simulink model "sm_stewart_platform"  (R2019b)
settings: Solver=ode45  StartTime=0.0  StopTime=450  MaxStep=0.2  RelTol=1e-3  EnableMultiTasking=on
model workspace (MAT data in the model file):
  g_density = 5
values from neighbouring files (symbols this model uses):
  B = base_points.Data(:,:,1)    [run_this_for_sim.m]
  base_radius = 0.75*100    (= 75)    [run_this_for_sim.m]
  desired_max_angle = 10    [run_this_for_sim.m]
  desired_max_x = 0.05    [run_this_for_sim.m]
  desired_max_y = desired_max_x    (= 0.05)    [run_this_for_sim.m]
  desired_max_z = 0.05    [run_this_for_sim.m]
  initial_integral_force = 200    [run_this_for_sim.m]
  leg_max = leg_min+0.3    (= 1.322)    [run_this_for_sim.m]
  leg_min = 1.022    [run_this_for_sim.m]
  leg_thickness = 75/1000    (= 0.075)    [run_this_for_sim.m]
  lower_leg_length = upper_leg_length    (= 0.511)    [run_this_for_sim.m]
  max_velocity = 0.15    [run_this_for_sim.m]
  P = platform_points.Data(:,:,1)    [run_this_for_sim.m]
  platform_radius = 0.75*base_radius    (= 56.25)    [run_this_for_sim.m]
  platform_thickness = 0.1/8    (= 0.0125)    [run_this_for_sim.m]
  trajectory_smoothing = 1/1.5    (= 0.666666666667)    [run_this_for_sim.m]
  upper_leg_length = dead_length/2    (= 0.511)    [run_this_for_sim.m]
  work_height = 1.2*100    (= 120)    [run_this_for_sim.m]
undefined symbols (not defined in the file or in its folder): nom_length, X, Z
libraries: sp_lib x18, nesl_utility x11, sm_lib x9, simulink x2
(part 4 of 10)

== system sm_stewart_platform/Reference Trajectory Generator6/Euler XYZ ==
  angles : Inport
  11 : Fcn  Expr=cos(u[2])*cos(u[3])
  12 : Fcn  Expr=-cos(u[2])*sin(u[3])
  13 : Fcn  Expr=sin(u[2])
  21 : Fcn  Expr=cos(u[3])*sin(u[2])*sin(u[1])+cos(u[1])*sin(u[3])
  22 : Fcn  Expr=cos(u[1])*cos(u[3]) - sin(u[1])*sin(u[2])*sin(u[3])
  23 : Fcn  Expr=-sin(u[1])*cos(u[2])
  31 : Fcn  Expr=sin(u[1])*sin(u[3]) - cos(u[1])*cos(u[3])*sin(u[2])
  32 : Fcn  Expr=cos(u[3])*sin(u[1])+cos(u[1])*sin(u[2])*sin(u[3])
  33 : Fcn  Expr=cos(u[1])*cos(u[2])
  Mux2 : Mux  Inputs=9
  Reshape 9x1->3x3 : Reshape  OutputDimensionality=Customize  OutputDimensions=[3,3]
  R : Outport  VectorParamsAs1DForOutWhenUnconnected=off
  wires:
  angles/1 -> 23/1, 33/1, 13/1, 32/1, 22/1, 12/1, 31/1, 21/1, 11/1
  33/1 -> Mux2/9
  23/1 -> Mux2/8
  13/1 -> Mux2/7
  32/1 -> Mux2/6
  22/1 -> Mux2/5
  12/1 -> Mux2/4
  31/1 -> Mux2/3
  21/1 -> Mux2/2
  11/1 -> Mux2/1
  Mux2/1 -> Reshape 9x1->3x3/1
  Reshape 9x1->3x3/1 -> R/1

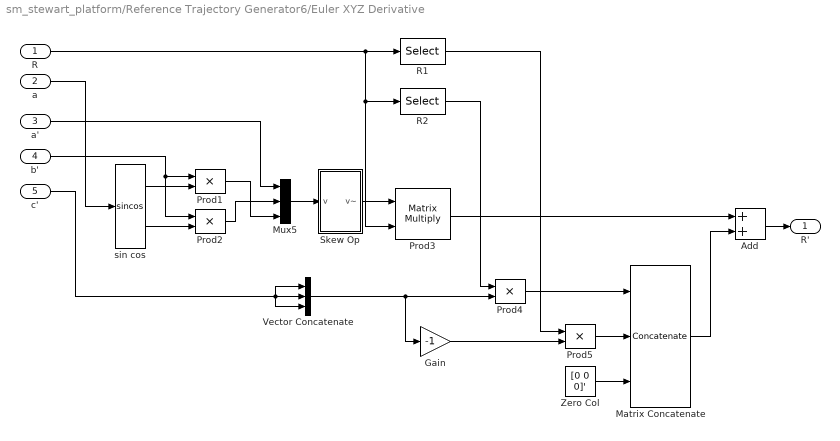
== system sm_stewart_platform/Reference Trajectory Generator6/Euler XYZ Derivative ==
  R : Inport
  a : Inport  Port=2
  a' : Inport  Port=3
  b' : Inport  Port=4
  c' : Inport  Port=5
  Add : Sum
  Gain : Gain  Gain=-1
  Matrix Concatenate : Concatenate  NumInputs=3  Mode=Multidimensional array  ConcatenateDimension=2
  Mux5 : Mux  Inputs=3
  Prod{1..2,4..5} (4 alike) : Product  RndMeth=Zero
  Prod3 : Product  Multiplication=Matrix(*)  RndMeth=Zero
  R1 : Selector  NumberOfDimensions=2  InputPortWidth=3  IndexOptions=Select all,Index vector (dialog)  Indices=[1 3],1  OutputSizes=1,1
  R2 : Selector  NumberOfDimensions=2  InputPortWidth=3  IndexOptions=Select all,Index vector (dialog)  Indices=[1 3],2  OutputSizes=1,1
  Skew Op : Subsystem
  Vector Concatenate : Concatenate  NumInputs=3  Mode=Multidimensional array
  Zero Col : Constant  Value=[0 0 0]'
  sin cos : Trigonometry  Operator=sincos
  R' : Outport  VectorParamsAs1DForOutWhenUnconnected=off
  wires:
  a/1 -> sin cos/1
  sin cos/1 -> Prod1/2
  sin cos/2 -> Prod2/2
  b'/1 -> Prod2/1, Prod1/1
  a'/1 -> Mux5/1
  Prod2/1 -> Mux5/2
  Prod1/1 -> Mux5/3
  Mux5/1 -> Skew Op/1(v)
  Vector Concatenate/1 -> Prod4/2, Gain/1
  R2/1 -> Prod4/1
  Gain/1 -> Prod5/2
  Zero Col/1 -> Matrix Concatenate/3
  Prod5/1 -> Matrix Concatenate/2
  Prod4/1 -> Matrix Concatenate/1
  R1/1 -> Prod5/1
  Prod3/1 -> Add/1
  Matrix Concatenate/1 -> Add/2
  Add/1 -> R'/1
  R/1 -> R1/1, Prod3/2, R2/1
  Skew Op/1(v~) -> Prod3/1
  c'/1 -> Vector Concatenate/2, Vector Concatenate/1, Vector Concatenate/3

== system sm_stewart_platform/Reference Trajectory Generator6/Rx sinusoid ==
  t : Inport
  Add : Sum  Inputs=|++
  Add2 : Sum  Inputs=++|
  amp1 : Gain  Gain=A
  amp2 : Gain  Gain=w*A*pi/180
  deg2rad : Gain  Gain=pi/180
  freq : Gain  Gain=w
  offset : Constant  Value=k  VectorParams1D=off
  phase : Constant  Value=p  VectorParams1D=off
  sin cos : Trigonometry  Operator=sincos
  f : Outport  VectorParamsAs1DForOutWhenUnconnected=off
  f' : Outport  Port=2  VectorParamsAs1DForOutWhenUnconnected=off
  wires:
  t/1 -> freq/1
  Add/1 -> deg2rad/1
  phase/1 -> Add/2
  amp2/1 -> f'/1
  Add2/1 -> f/1
  offset/1 -> Add2/1
  sin cos/1 -> amp1/1
  sin cos/2 -> amp2/1
  amp1/1 -> Add2/2
  freq/1 -> Add/1
  deg2rad/1 -> sin cos/1

== system sm_stewart_platform/Reference Trajectory Generator6/Ry sinusoid ==
  t : Inport
  Add : Sum  Inputs=|++
  Add2 : Sum  Inputs=++|
  amp1 : Gain  Gain=A
  amp2 : Gain  Gain=w*A*pi/180
  deg2rad : Gain  Gain=pi/180
  freq : Gain  Gain=w
  offset : Constant  Value=k  VectorParams1D=off
  phase : Constant  Value=p  VectorParams1D=off
  sin cos : Trigonometry  Operator=sincos
  f : Outport  VectorParamsAs1DForOutWhenUnconnected=off
  f' : Outport  Port=2  VectorParamsAs1DForOutWhenUnconnected=off
  wires:
  t/1 -> freq/1
  Add/1 -> deg2rad/1
  phase/1 -> Add/2
  amp2/1 -> f'/1
  Add2/1 -> f/1
  offset/1 -> Add2/1
  sin cos/1 -> amp1/1
  sin cos/2 -> amp2/1
  amp1/1 -> Add2/2
  freq/1 -> Add/1
  deg2rad/1 -> sin cos/1

== system sm_stewart_platform/Reference Trajectory Generator6/Rz sinusoid ==
  t : Inport
  Add : Sum  Inputs=|++
  Add2 : Sum  Inputs=++|
  amp1 : Gain  Gain=A
  amp2 : Gain  Gain=w*A*pi/180
  deg2rad : Gain  Gain=pi/180
  freq : Gain  Gain=w
  offset : Constant  Value=k  VectorParams1D=off
  phase : Constant  Value=p  VectorParams1D=off
  sin cos : Trigonometry  Operator=sincos
  f : Outport  VectorParamsAs1DForOutWhenUnconnected=off
  f' : Outport  Port=2  VectorParamsAs1DForOutWhenUnconnected=off
  wires:
  t/1 -> freq/1
  Add/1 -> deg2rad/1
  phase/1 -> Add/2
  amp2/1 -> f'/1
  Add2/1 -> f/1
  offset/1 -> Add2/1
  sin cos/1 -> amp1/1
  sin cos/2 -> amp2/1
  amp1/1 -> Add2/2
  freq/1 -> Add/1
  deg2rad/1 -> sin cos/1

== system sm_stewart_platform/Reference Trajectory Generator6/dx sinusoid ==
  t : Inport
  Add : Sum  Inputs=|++
  Add2 : Sum  Inputs=++|
  amp1 : Gain  Gain=A
  amp2 : Gain  Gain=w*A*pi/180
  deg2rad : Gain  Gain=pi/180
  freq : Gain  Gain=w
  offset : Constant  Value=k  VectorParams1D=off
  phase : Constant  Value=p  VectorParams1D=off
  sin cos : Trigonometry  Operator=sincos
  f : Outport  VectorParamsAs1DForOutWhenUnconnected=off
  f' : Outport  Port=2  VectorParamsAs1DForOutWhenUnconnected=off
  wires:
  t/1 -> freq/1
  Add/1 -> deg2rad/1
  phase/1 -> Add/2
  amp2/1 -> f'/1
  Add2/1 -> f/1
  offset/1 -> Add2/1
  sin cos/1 -> amp1/1
  sin cos/2 -> amp2/1
  amp1/1 -> Add2/2
  freq/1 -> Add/1
  deg2rad/1 -> sin cos/1

== system sm_stewart_platform/Reference Trajectory Generator6/dy sinusoid ==
  t : Inport
  Add : Sum  Inputs=|++
  Add2 : Sum  Inputs=++|
  amp1 : Gain  Gain=A
  amp2 : Gain  Gain=w*A*pi/180
  deg2rad : Gain  Gain=pi/180
  freq : Gain  Gain=w
  offset : Constant  Value=k  VectorParams1D=off
  phase : Constant  Value=p  VectorParams1D=off
  sin cos : Trigonometry  Operator=sincos
  f : Outport  VectorParamsAs1DForOutWhenUnconnected=off
  f' : Outport  Port=2  VectorParamsAs1DForOutWhenUnconnected=off
  wires:
  t/1 -> freq/1
  Add/1 -> deg2rad/1
  phase/1 -> Add/2
  amp2/1 -> f'/1
  Add2/1 -> f/1
  offset/1 -> Add2/1
  sin cos/1 -> amp1/1
  sin cos/2 -> amp2/1
  amp1/1 -> Add2/2
  freq/1 -> Add/1
  deg2rad/1 -> sin cos/1

== system sm_stewart_platform/Reference Trajectory Generator6/dz sinusoid ==
  t : Inport
  Add : Sum  Inputs=|++
  Add2 : Sum  Inputs=++|
  amp1 : Gain  Gain=A
  amp2 : Gain  Gain=w*A*pi/180
  deg2rad : Gain  Gain=pi/180
  freq : Gain  Gain=w
  offset : Constant  Value=k  VectorParams1D=off
  phase : Constant  Value=p  VectorParams1D=off
  sin cos : Trigonometry  Operator=sincos
  f : Outport  VectorParamsAs1DForOutWhenUnconnected=off
  f' : Outport  Port=2  VectorParamsAs1DForOutWhenUnconnected=off
  wires:
  t/1 -> freq/1
  Add/1 -> deg2rad/1
  phase/1 -> Add/2
  amp2/1 -> f'/1
  Add2/1 -> f/1
  offset/1 -> Add2/1
  sin cos/1 -> amp1/1
  sin cos/2 -> amp2/1
  amp1/1 -> Add2/2
  freq/1 -> Add/1
  deg2rad/1 -> sin cos/1

== system sm_stewart_platform/Reference Trajectory Generator6/manual ==
  Constant : Constant
  Constant1 : Constant  Value=work_height
  Derivative : Derivative
  Slider Gain : simulink/Math Operations/Slider Gain  gain=-45.0  low=-250  high=250
  Sum : Sum  Inputs=|++
  x : Outport  VectorParamsAs1DForOutWhenUnconnected=off
  x' : Outport  Port=2  VectorParamsAs1DForOutWhenUnconnected=off
  wires:
  Sum/1 -> Derivative/1, x/1
  Constant/1 -> Slider Gain/1
  Derivative/1 -> x'/1
  Slider Gain/1 -> Sum/1
  Constant1/1 -> Sum/2

== system sm_stewart_platform/Stewart Platform System/Controller ==
  act_pos : Inport
  act_vel : Inport  Port=2
  des_pos : Inport  Port=3
  des_vel : Inport  Port=4
  D : Gain  Gain=Kd  SaturateOnIntegerOverflow=on  OutDataTypeStr=Inherit: Same as input  ParamDataTypeStr=Inherit: Same as input
  Gain : Gain
  I : Gain  Gain=Ki  SaturateOnIntegerOverflow=on  OutDataTypeStr=Inherit: Same as input  ParamDataTypeStr=Inherit: Same as input
  Integrator : Integrator  InitialCondition=initial_integral_force/Ki(1)
  P : Gain  Gain=Kp  SaturateOnIntegerOverflow=on  OutDataTypeStr=Inherit: Same as input  ParamDataTypeStr=Inherit: Same as input
  PID : Scope  NumInputPorts=3
  Sum : Sum  Inputs=-+|  SaturateOnIntegerOverflow=on  InputSameDT=on  OutDataTypeStr=Inherit: Same as first input
  Sum1 : Sum  Inputs=+++  SaturateOnIntegerOverflow=on  InputSameDT=on  OutDataTypeStr=Inherit: Same as first input
  Sum2 : Sum  Inputs=-+|  SaturateOnIntegerOverflow=on  InputSameDT=on  OutDataTypeStr=Inherit: Same as first input
  force : Outport  VectorParamsAs1DForOutWhenUnconnected=off
  wires:
  Sum/1 -> Integrator/1, P/1
  P/1 -> PID/1, Sum1/1
  act_pos/1 -> Sum/1
  des_pos/1 -> Sum/2
  act_vel/1 -> Sum2/1
  des_vel/1 -> Gain/1
  D/1 -> PID/3, Sum1/3
  I/1 -> PID/2, Sum1/2
  Sum1/1 -> force/1
  Integrator/1 -> I/1
  Gain/1 -> Sum2/2
  Sum2/1 -> D/1

== system sm_stewart_platform/Stewart Platform System/Ideal PID ==
  act_pos : Inport
  act_vel : Inport  Port=2
  des_pos : Inport  Port=3
  des_vel : Inport  Port=4
  D : Gain  Gain=Kd  SaturateOnIntegerOverflow=on  OutDataTypeStr=Inherit: Same as input  ParamDataTypeStr=Inherit: Same as input
  Gain : Gain
  I : Gain  Gain=1/Ki  SaturateOnIntegerOverflow=on  OutDataTypeStr=Inherit: Same as input  ParamDataTypeStr=Inherit: Same as input
  Ideal PID : Scope  NumInputPorts=3
  Integrator : Integrator  InitialCondition=initial_integral_force*Ki(1)/Kp(1)
  P{,1..3} (4 alike) : Gain  Gain=Kp  SaturateOnIntegerOverflow=on  OutDataTypeStr=Inherit: Same as input  ParamDataTypeStr=Inherit: Same as input
  Sum : Sum  Inputs=-+|  SaturateOnIntegerOverflow=on  InputSameDT=on  OutDataTypeStr=Inherit: Same as first input
  Sum1 : Sum  Inputs=+++  SaturateOnIntegerOverflow=on  InputSameDT=on  OutDataTypeStr=Inherit: Same as first input
  Sum2 : Sum  Inputs=-+|  SaturateOnIntegerOverflow=on  InputSameDT=on  OutDataTypeStr=Inherit: Same as first input
  force : Outport  VectorParamsAs1DForOutWhenUnconnected=off
  wires:
  Sum/1 -> P1/1, Sum1/1, Integrator/1
  act_pos/1 -> Sum/1
  des_pos/1 -> Sum/2
  act_vel/1 -> Sum2/1
  des_vel/1 -> Gain/1
  Integrator/1 -> I/1
  Gain/1 -> Sum2/2
  P/1 -> force/1
  I/1 -> P2/1, Sum1/2
  D/1 -> P3/1, Sum1/3
  Sum1/1 -> P/1
  P1/1 -> Ideal PID/1
  P2/1 -> Ideal PID/2
  P3/1 -> Ideal PID/3
  Sum2/1 -> D/1

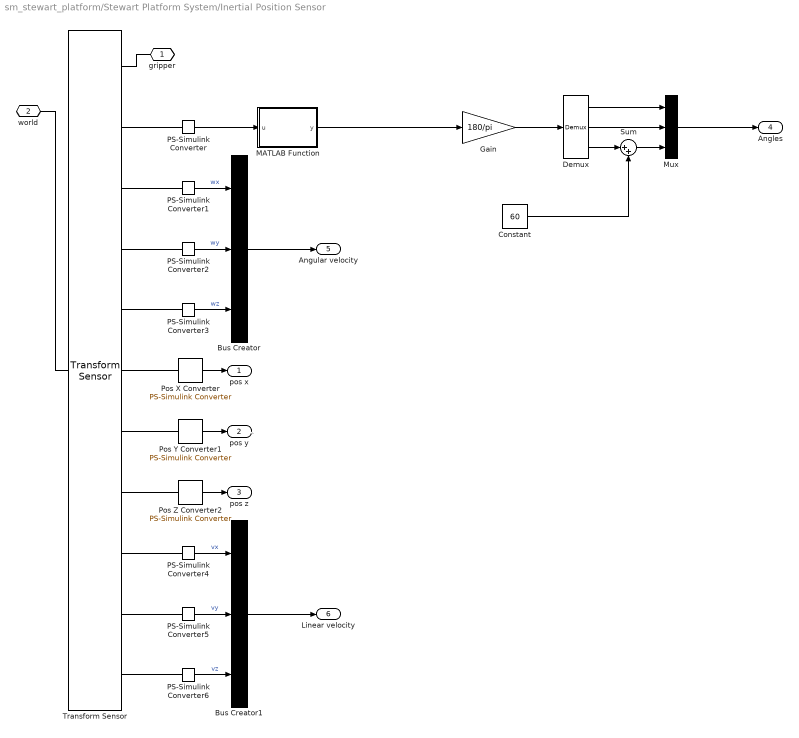
== system sm_stewart_platform/Stewart Platform System/Inertial Position Sensor ==
  note: `
  Bus Creator : BusCreator  Inputs=3
  Bus Creator1 : BusCreator  Inputs=3
  Constant : Constant  Value=60
  Demux : Demux  Outputs=3
  Gain : Gain  Gain=180/pi
  MATLAB Function : MATLAB Function  TreatAsAtomicUnit=on
  Mux : Mux  Inputs=3
  PS-Simulink Converter : nesl_utility/PS-Simulink Converter  PhysicalDomain=network_engine_domain  SubClassName=ps_output  LeftPortType=input  RightPortType=output  PseudoPeriodic=off  Frequencies=[]  Unit=1  AffineConversion=off
  PS-Simulink Converter1 : nesl_utility/PS-Simulink Converter  PhysicalDomain=network_engine_domain  SubClassName=ps_output  LeftPortType=input  RightPortType=output  PseudoPeriodic=off  Frequencies=[]  Unit=deg/s  AffineConversion=off
  PS-Simulink Converter2 : nesl_utility/PS-Simulink Converter  PhysicalDomain=network_engine_domain  SubClassName=ps_output  LeftPortType=input  RightPortType=output  PseudoPeriodic=off  Frequencies=[]  Unit=deg/s  AffineConversion=off
  PS-Simulink Converter3 : nesl_utility/PS-Simulink Converter  PhysicalDomain=network_engine_domain  SubClassName=ps_output  LeftPortType=input  RightPortType=output  PseudoPeriodic=off  Frequencies=[]  Unit=deg/s  AffineConversion=off
  PS-Simulink Converter4 : nesl_utility/PS-Simulink Converter  PhysicalDomain=network_engine_domain  SubClassName=ps_output  LeftPortType=input  RightPortType=output  PseudoPeriodic=off  Frequencies=[]  Unit=m/s  AffineConversion=off
  PS-Simulink Converter5 : nesl_utility/PS-Simulink Converter  PhysicalDomain=network_engine_domain  SubClassName=ps_output  LeftPortType=input  RightPortType=output  PseudoPeriodic=off  Frequencies=[]  Unit=m/s  AffineConversion=off
  PS-Simulink Converter6 : nesl_utility/PS-Simulink Converter  PhysicalDomain=network_engine_domain  SubClassName=ps_output  LeftPortType=input  RightPortType=output  PseudoPeriodic=off  Frequencies=[]  Unit=m/s  AffineConversion=off
  Pos X Converter : nesl_utility/PS-Simulink Converter  PhysicalDomain=network_engine_domain  SubClassName=ps_output  LeftPortType=input  RightPortType=output  PseudoPeriodic=off  Frequencies=[]  Unit=cm  AffineConversion=off
  Pos Y Converter1 : nesl_utility/PS-Simulink Converter  PhysicalDomain=network_engine_domain  SubClassName=ps_output  LeftPortType=input  RightPortType=output  PseudoPeriodic=off  Frequencies=[]  Unit=cm  AffineConversion=off
  Pos Z Converter2 : nesl_utility/PS-Simulink Converter  PhysicalDomain=network_engine_domain  SubClassName=ps_output  LeftPortType=input  RightPortType=output  PseudoPeriodic=off  Frequencies=[]  Unit=cm  AffineConversion=off
  Sum : Sum  Inputs=|++
  Transform Sensor : sm_lib/Frames and Transforms/Transform Sensor  MeasurementFrame=World  SenseAngle=off  SenseAxis=off  SenseAngle1=off  SenseAngle2=off  SenseAngle3=off  SenseQ=on  SenseR=off  SenseOmegaX=on  SenseOmegaY=on  SenseOmegaZ=on  SenseOmega1=off  SenseOmega2=off  SenseOmega3=off  SenseQDot=off  SenseRDot=off  SenseAlphaX=off  SenseAlphaY=off  SenseAlphaZ=off  SenseAlpha1=off  SenseAlpha2=off  SenseAlpha3=off  SenseQDDot=off  SenseRDDot=off  SenseX=on  SenseY=on  SenseZ=on  SenseRad=off  SenseAzim=off  SenseDist=off  SenseInc=off  SenseXDot=on  SenseYDot=on  SenseZDot=on  SenseRadDot=off  SenseAzimDot=off  SenseDistDot=off  SenseIncDot=off  SenseXDDot=off  SenseYDDot=off  SenseZDDot=off  SenseRadDDot=off  SenseAzimDDot=off  SenseDistDDot=off  SenseIncDDot=off
  gripper : PMIOPort  Side=Left
  world : PMIOPort  Port=2  Side=Left
  pos x : Outport  VectorParamsAs1DForOutWhenUnconnected=off
  pos y : Outport  Port=2  VectorParamsAs1DForOutWhenUnconnected=off
  pos z : Outport  Port=3  VectorParamsAs1DForOutWhenUnconnected=off
  Angles : Outport  Port=4  VectorParamsAs1DForOutWhenUnconnected=off
  Angular velocity : Outport  Port=5  VectorParamsAs1DForOutWhenUnconnected=off
  Linear velocity : Outport  Port=6  VectorParamsAs1DForOutWhenUnconnected=off
  wires:
  Pos Z Converter2/1 -> pos z/1
  Pos Y Converter1/1 -> pos y/1
  Pos X Converter/1 -> pos x/1
  PS-Simulink Converter/1 -> MATLAB Function/1(u)
  MATLAB Function/1(y) -> Gain/1
  Gain/1 -> Demux/1
  Demux/1 -> Mux/1
  Demux/2 -> Mux/2
  Mux/1 -> Angles/1
  Demux/3 -> Sum/1
  Sum/1 -> Mux/3
  Constant/1 -> Sum/2
  PS-Simulink Converter1/1 -> Bus Creator/1  "wx"
  PS-Simulink Converter2/1 -> Bus Creator/2  "wy"
  PS-Simulink Converter3/1 -> Bus Creator/3  "wz"
  PS-Simulink Converter4/1 -> Bus Creator1/1  "vx"
  PS-Simulink Converter6/1 -> Bus Creator1/3  "vz"
  PS-Simulink Converter5/1 -> Bus Creator1/2  "vy"
  Bus Creator/1 -> Angular velocity/1
  Bus Creator1/1 -> Linear velocity/1
  connections:
  world/RConn1 -- Transform Sensor/LConn1
  gripper/RConn1 -- Transform Sensor/RConn1
  PS-Simulink Converter/LConn1 -- Transform Sensor/RConn2
  Pos X Converter/LConn1 -- Transform Sensor/RConn6
  Transform Sensor/RConn7 -- Pos Y Converter1/LConn1
  Transform Sensor/RConn8 -- Pos Z Converter2/LConn1
  PS-Simulink Converter1/LConn1 -- Transform Sensor/RConn3
  Transform Sensor/RConn4 -- PS-Simulink Converter2/LConn1
  PS-Simulink Converter3/LConn1 -- Transform Sensor/RConn5
  Transform Sensor/RConn9 -- PS-Simulink Converter4/LConn1
  Transform Sensor/RConn10 -- PS-Simulink Converter5/LConn1
  Transform Sensor/RConn11 -- PS-Simulink Converter6/LConn1

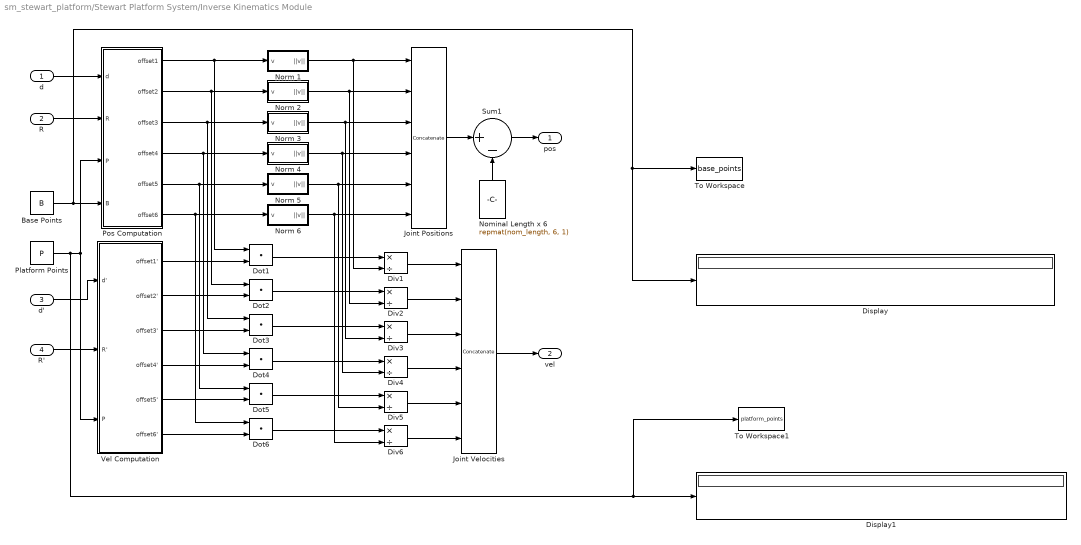
== system sm_stewart_platform/Stewart Platform System/Inverse Kinematics Module ==
  d : Inport
  R : Inport  Port=2
  d' : Inport  Port=3
  R' : Inport  Port=4
  Base Points : Constant  Value=B
  Display : Display
  Display1 : Display
  Div{1..6} (6 alike) : Product  Inputs=*/
  Dot{1..6} (6 alike) : DotProduct  OutDataTypeStr=Inherit: Inherit via internal rule
  Joint Positions : Concatenate  NumInputs=6  Mode=Multidimensional array
  Joint Velocities : Concatenate  NumInputs=6  Mode=Multidimensional array
  Nominal Length x 6 : Constant  Value=repmat(nom_length, 6, 1)
  Norm 1 : Subsystem
  Norm 2 : Subsystem
  Norm 3 : Subsystem
  Norm 4 : Subsystem
  Norm 5 : Subsystem
  Norm 6 : Subsystem
  Platform Points : Constant  Value=P
  Pos Computation : Subsystem
  Sum1 : Sum  Inputs=|+-
  To Workspace : ToWorkspace  VariableName=base_points  SaveFormat=Timeseries  SampleTime=-1
  To Workspace1 : ToWorkspace  VariableName=platform_points  SaveFormat=Timeseries  SampleTime=-1
  Vel Computation : Subsystem
  pos : Outport  VectorParamsAs1DForOutWhenUnconnected=off
  vel : Outport  Port=2  VectorParamsAs1DForOutWhenUnconnected=off
  wires:
  Joint Positions/1 -> Sum1/1
  Nominal Length x 6/1 -> Sum1/2
  Sum1/1 -> pos/1
  d/1 -> Pos Computation/1(d)
  R/1 -> Pos Computation/2(R)
  Base Points/1 -> To Workspace/1, Display/1, Pos Computation/4(B)
  Platform Points/1 -> To Workspace1/1, Display1/1, Vel Computation/3(P), Pos Computation/3(P)
  Pos Computation/4(offset4) -> Norm 4/1(v), Dot4/1
  Pos Computation/3(offset3) -> Norm 3/1(v), Dot3/1
  Pos Computation/2(offset2) -> Norm 2/1(v), Dot2/1
  Pos Computation/1(offset1) -> Norm 1/1(v), Dot1/1
  Pos Computation/5(offset5) -> Norm 5/1(v), Dot5/1
  Pos Computation/6(offset6) -> Norm 6/1(v), Dot6/1
  Norm 1/1(||v||) -> Joint Positions/1, Div1/2
  Norm 6/1(||v||) -> Joint Positions/6, Div6/2
  Norm 2/1(||v||) -> Joint Positions/2, Div2/2
  Norm 3/1(||v||) -> Joint Positions/3, Div3/2
  Norm 4/1(||v||) -> Joint Positions/4, Div4/2
  Norm 5/1(||v||) -> Joint Positions/5, Div5/2
  Vel Computation/3(offset3') -> Dot3/2
  Vel Computation/4(offset4') -> Dot4/2
  Vel Computation/2(offset2') -> Dot2/2
  Vel Computation/5(offset5') -> Dot5/2
  Vel Computation/6(offset6') -> Dot6/2
  d'/1 -> Vel Computation/1(d')
  Dot2/1 -> Div2/1
  Dot6/1 -> Div6/1
  Dot5/1 -> Div5/1
  Dot4/1 -> Div4/1
  Dot3/1 -> Div3/1
  Div1/1 -> Joint Velocities/1
  Div2/1 -> Joint Velocities/2
  Div6/1 -> Joint Velocities/6
  Div3/1 -> Joint Velocities/3
  Div4/1 -> Joint Velocities/4
  Div5/1 -> Joint Velocities/5
  Joint Velocities/1 -> vel/1
  R'/1 -> Vel Computation/2(R')
  Vel Computation/1(offset1') -> Dot1/2
  Dot1/1 -> Div1/1

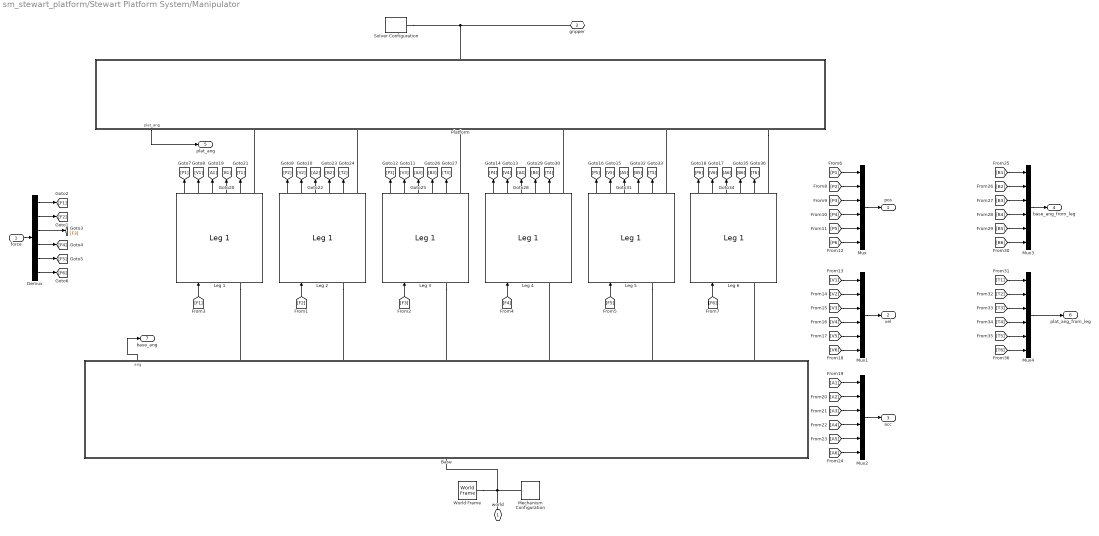
== system sm_stewart_platform/Stewart Platform System/Manipulator ==
  force : Inport
  Base : Subsystem  AncestorBlock=sm_stewart_platform_lib/Hexagon Plate  mask(Hexagon Plate){kind=base, hex_rad=base_rad, hex_thick=base_thick, hex_skew=hex_skew, flange_sep=2 * leg_rad * cos(pi/6) - flange_thick, flange_len=flange_len, flange_width=flange_width, flange_thick=flange_thick, diffuse=[0.4 0.3 0.2 0.5], specular=[0 0 0], shininess=10}
      mask prompts: hex_rad "Hexagon Radius (cm)"; hex_thick "Hexagon Thickness (cm)"; hex_skew "Hexagon Skew"; flange_sep "Flange Separation (cm)"; flange_len "Flange Length (cm)"; flange_width "Flange Width (cm)"; flange_thick "Flange Thickness (cm)"; diffuse "Diffuse (rgba)"; specular "Specular (rgba)"
      mask help:
      | Models a rigid body formed by attaching six couplings to the corners of a skewed hexagon.
      |
      | There are two hexagon plates in a Stewart platform manipulator: one forming the grounded base, and the other forming the moveable platform.  Six legs connect the corresponding couplings of these two plates.  Both plates are modeled with this block.
      mask init:
      | % Set up a value equal to 0 or 1 based on whether
      | % this is the base or platform, respectively.  This value
      | % is used in the computations of certain variables and
      | % transforms that differ for the two types of hexagon plates.
      | if (kind == 1)
      |     kind_val = 0;  % Value for base
      | else
      |     kind_val = 1;  % Value for platform
      | end
      mask Help:
      | A <em>Hexagon Plate</em> models a rigid body formed by attaching six couplings to the corners of a skewed hexagon.
      | 
      | There are two hexagon plates in a Stewart platform manipulator: one forming the grounded base, and the other forming the moveable platform.  Six legs connect the corresponding couplings of these two plates.  Both plates are modeled with this block.
      | 
      | <h3>Skewed Hexagons</h3>
      | 
      | The main part of a hexagon plate is a </em>skewed hexagon</em>.  This is short hexagonal prism.  The cross section is based on a regular hexagon, but with the vertices perturbed according to the skew factor, a real value in the range (-0.5, +0.5).
      | 
      | The vertices of a skewed hexagon always lie on a circle centered at the origin. The ith vertex (i = 1, 2, ..., 6) is located at the intersection of the ray at angle theta_i with this circle, where theta_i is given by
      | 
      | theta_i = [ i - 1 + (-1)^(i - 1) s ] * pi/3  radians,
      | 
      | where s is the skew factor.  A skew factor of zero produces vertices around the circle at angles 0, pi/3, 2/3 pi, pi, 4/3 pi, 5/3 pi.  In other words, the vertices form a regular hexagon.
      | 
      | As the skew factor increase in magnitude, the hexagon vertices are shifted so that the shape becomes more and more triangular, as pairs of vertices approach each another.  Three of the sides of the hexagon grow longer as the other three grow shorter.  Regardless of the skew factor, the skewed hexagon exhibits 3-fold symmetry.  It exhibits 6-fold symmetry for a zero skew factor only.  When the skew factor is +/- 1, pairs of vertices overlap and the cross section becomes an equilateral triangle; this configuration is degenerate and not allowed.
      | 
      | A skew factor of -s produces the same shape as a skew factor of +s, except that the three side that lengthen under a skew factor of +s shrink under a skew factor of -s, and vice versa.  For a hexagonal plate, this affects the way couplings are placed on the hexagon.  If the skew factor is positive, the couplings are placed along the long sides of the hexagon; if the skew factor is negative, the couplings are placed along the short sides.
      | 
      | <h3>Geometry</h3>
      | 
      | The <em>Geom</em> tab parameters specify the geometry of the hexagon plate.
      | 
      | <ul>
      | 
      | <li> <b>Kind</b> An enumerated parameter with possible values of <em>base</em> or <em>platform</em>.  This affects some computations that are slightly different for the two types of hexagon plates in a Stewart platform.  The differences stem from two reasons.  First, the couplings appear on the top side of the base plate but on the underside of the platform plate.  Second, the couplings indices on the platform plate are offset by one (modulo 6) relative to the coupling indices on the base plate.  This causes the legs of the platform to lean in directions tangential to the edges of the base and platform plates, which adds stability to the manipulator.
      | 
      | <li> <b>Hexagon Radius</b> The radius of the circle on which the vertices of the hexagonal cross section lie.
      | 
      | <li> <b>Hexagon Thickness</b> The thickness (length) of the hexagonal prism forming the main part of the hexagon plate.
      | 
      | <li> <b>Hexagon Skew</b> The skew factor of the hexagonal cross section, in the range (-0.5, +0.5).  See <em>Skewed Hexagons</em> above for details.
      | 
      | </ul>
      | 
      | <h3>Flanges</h3>
      | 
      | The <em>Flanges</em> tab parameters specify the geometry of the flanges of the six couplings of the hexagonal plate.
      | 
      | <ul>
      | 
      | <li> <b>Flange Separation</b> The flange separation of the couplings of the hexagon plate.  See <em>Coupling</em> block for details.
      | 
      | <li> <b>Flange Length</b> The length of the coupling flanges. See <em>Coupling</em> block for details.
      | 
      | <li> <b>Flange Width</b> The width of the coupling flanges. See <em>Coupling</em> block for details.
      | 
      | <li> <b>Flange Thickness</b> The thickness of the coupling flanges. See <em>Coupling</em> block for details.
      | 
      | </ul>
      | 
      | <h3>Visualization</h3>
      | 
      | The <em>Graphics</em> tab parameters specify the visualization aspects of the hexagon plate.  The skewed hexagon and all six couplings share the same visual properties.
      | 
      | <ul>
      | 
      | <li> <b>Diffuse</b> The diffuse color of the hexagon plate.  This is an RGB 3-vector or an RGBA 4-vector with all components in the range [0, 1].
      | 
      | <li> <b>Specular</b> The specular color of the hexagon plate.  This is an RGB 3-vector or an RGBA 4-vector with all components in the range [0, 1].
      | 
      | <li> <b>Shininess</b> The shininess of the hexagon plate.  This is a scalar value in the range [0, 128].
      | 
      | </ul>
      | 
      | 
      | <h3>Ports</h3>
      | 
      | <ul>
      | 
      | <li> <b>ref</b> Reference frame of the hexagon plate.  The origin of this frame is located at the center of the skewed hexagon prism.  For a base plate, this frame is typically attached to ground or a supporting body.  For the platform plate, this frame is used to define an attachment point for a payload or end effector.
      | 
      | <li> <b>leg1, ..., leg6</b> Attachment frames for the six legs of the Stewart platform.  Each leg is attached to one of these six frames through one of its crosspieces.  When all six legs are connected to both hexagon plates in this manner, the result is a kinematically valid Stewart platform manipulator.
      | 
      | </ul>
      mask TypeOptions kind: base | platform
      mask Display:
      | image(imread('sm_stewart_platform_hexagonplate.png'))
      | color('white')
      | port_label('LConn', 1, 'ref')
      | port_label('RConn', 1, 'leg1')
      | port_label('RConn', 2, 'leg2')
      | port_label('RConn', 3, 'leg3')
      | port_label('RConn', 4, 'leg4')
      | port_label('RConn', 5, 'leg5')
      | port_label('RConn', 6, 'leg6')
  Demux : Demux  Outputs=6
  Leg {1..6} (6 alike) : sp_lib/Leg 1  upper_leg_len=upper_leg_len  lower_leg_len=lower_leg_len  rad=leg_rad  collar_thick=collar_thick  flange_len=flange_len  flange_width=flange_width  flange_thick=flange_thick  asm_offset=lengths(1)
      settings: SourceProductName=Simscape Multibody  SourceProductBaseCode=MS
  Mechanism Configuration : sm_lib/Utilities/Mechanism Configuration  UniformGravity=Constant  GravityVector=[0 0 -9.81]  GravityUnits=m/s^2  LinearizationDelta=0.001
  Mux{,1..4} (5 alike) : Mux  Inputs=6
  Platform : Subsystem  AncestorBlock=sm_stewart_platform_lib/Hexagon Plate  mask(Hexagon Plate){kind=platform, hex_rad=platform_rad, hex_thick=platform_thick, hex_skew=hex_skew, flange_sep=2 * leg_rad * cos(pi/6) - flange_thick, flange_len=flange_len, flange_width=flange_width, flange_thick=flange_thick, diffuse=[.7 .7 .3 0.75], specular=[.7 .7 .3 0.75], shininess=90}
      mask prompts: hex_rad "Hexagon Radius (cm)"; hex_thick "Hexagon Thickness (cm)"; hex_skew "Hexagon Skew"; flange_sep "Flange Separation (cm)"; flange_len "Flange Length (cm)"; flange_width "Flange Width (cm)"; flange_thick "Flange Thickness (cm)"; diffuse "Diffuse (rgba)"; specular "Specular (rgba)"
      mask help:
      | Models a rigid body formed by attaching six couplings to the corners of a skewed hexagon.
      |
      | There are two hexagon plates in a Stewart platform manipulator: one forming the grounded base, and the other forming the moveable platform.  Six legs connect the corresponding couplings of these two plates.  Both plates are modeled with this block.
      mask init: same as sm_stewart_platform/Stewart Platform System/Manipulator/Base
      mask Help:
      | A <em>Hexagon Plate</em> models a rigid body formed by attaching six couplings to the corners of a skewed hexagon.
      | 
      | There are two hexagon plates in a Stewart platform manipulator: one forming the grounded base, and the other forming the moveable platform.  Six legs connect the corresponding couplings of these two plates.  Both plates are modeled with this block.
      | 
      | <h3>Skewed Hexagons</h3>
      | 
      | The main part of a hexagon plate is a </em>skewed hexagon</em>.  This is short hexagonal prism.  The cross section is based on a regular hexagon, but with the vertices perturbed according to the skew factor, a real value in the range (-0.5, +0.5).
      | 
      | The vertices of a skewed hexagon always lie on a circle centered at the origin. The ith vertex (i = 1, 2, ..., 6) is located at the intersection of the ray at angle theta_i with this circle, where theta_i is given by
      | 
      | theta_i = [ i - 1 + (-1)^(i - 1) s ] * pi/3  radians,
      | 
      | where s is the skew factor.  A skew factor of zero produces vertices around the circle at angles 0, pi/3, 2/3 pi, pi, 4/3 pi, 5/3 pi.  In other words, the vertices form a regular hexagon.
      | 
      | As the skew factor increase in magnitude, the hexagon vertices are shifted so that the shape becomes more and more triangular, as pairs of vertices approach each another.  Three of the sides of the hexagon grow longer as the other three grow shorter.  Regardless of the skew factor, the skewed hexagon exhibits 3-fold symmetry.  It exhibits 6-fold symmetry for a zero skew factor only.  When the skew factor is +/- 1, pairs of vertices overlap and the cross section becomes an equilateral triangle; this configuration is degenerate and not allowed.
      | 
      | A skew factor of -s produces the same shape as a skew factor of +s, except that the three side that lengthen under a skew factor of +s shrink under a skew factor of -s, and vice versa.  For a hexagonal plate, this affects the way couplings are placed on the hexagon.  If the skew factor is positive, the couplings are placed along the long sides of the hexagon; if the skew factor is negative, the couplings are placed along the short sides.
      | 
      | <h3>Geometry</h3>
      | 
      | The <em>Geom</em> tab parameters specify the geometry of the hexagon plate.
      | 
      | <ul>
      | 
      | <li> <b>Kind</b> An enumerated parameter with possible values of <em>base</em> or <em>platform</em>.  This affects some computations that are slightly different for the two types of hexagon plates in a Stewart platform.  The differences stem from two reasons.  First, the couplings appear on the top side of the base plate but on the underside of the platform plate.  Second, the couplings indices on the platform plate are offset by one (modulo 6) relative to the coupling indices on the base plate.  This causes the legs of the platform to lean in directions tangential to the edges of the base and platform plates, which adds stability to the manipulator.
      | 
      | <li> <b>Hexagon Radius</b> The radius of the circle on which the vertices of the hexagonal cross section lie.
      | 
      | <li> <b>Hexagon Thickness</b> The thickness (length) of the hexagonal prism forming the main part of the hexagon plate.
      | 
      | <li> <b>Hexagon Skew</b> The skew factor of the hexagonal cross section, in the range (-0.5, +0.5).  See <em>Skewed Hexagons</em> above for details.
      | 
      | </ul>
      | 
      | <h3>Flanges</h3>
      | 
      | The <em>Flanges</em> tab parameters specify the geometry of the flanges of the six couplings of the hexagonal plate.
      | 
      | <ul>
      | 
      | <li> <b>Flange Separation</b> The flange separation of the couplings of the hexagon plate.  See <em>Coupling</em> block for details.
      | 
      | <li> <b>Flange Length</b> The length of the coupling flanges. See <em>Coupling</em> block for details.
      | 
      | <li> <b>Flange Width</b> The width of the coupling flanges. See <em>Coupling</em> block for details.
      | 
      | <li> <b>Flange Thickness</b> The thickness of the coupling flanges. See <em>Coupling</em> block for details.
      | 
      | </ul>
      | 
      | <h3>Visualization</h3>
      | 
      | The <em>Graphics</em> tab parameters specify the visualization aspects of the hexagon plate.  The skewed hexagon and all six couplings share the same visual properties.
      | 
      | <ul>
      | 
      | <li> <b>Diffuse</b> The diffuse color of the hexagon plate.  This is an RGB 3-vector or an RGBA 4-vector with all components in the range [0, 1].
      | 
      | <li> <b>Specular</b> The specular color of the hexagon plate.  This is an RGB 3-vector or an RGBA 4-vector with all components in the range [0, 1].
      | 
      | <li> <b>Shininess</b> The shininess of the hexagon plate.  This is a scalar value in the range [0, 128].
      | 
      | </ul>
      | 
      | 
      | <h3>Ports</h3>
      | 
      | <ul>
      | 
      | <li> <b>ref</b> Reference frame of the hexagon plate.  The origin of this frame is located at the center of the skewed hexagon prism.  For a base plate, this frame is typically attached to ground or a supporting body.  For the platform plate, this frame is used to define an attachment point for a payload or end effector.
      | 
      | <li> <b>leg1, ..., leg6</b> Attachment frames for the six legs of the Stewart platform.  Each leg is attached to one of these six frames through one of its crosspieces.  When all six legs are connected to both hexagon plates in this manner, the result is a kinematically valid Stewart platform manipulator.
      | 
      | </ul>
      mask TypeOptions kind: base | platform
      mask DialogControl ParameterTabVar0 Prompt: Geom
      mask DialogControl ParameterTabVar01 Prompt: Flanges
      mask DialogControl ParameterTabVar012 Prompt: Graphics
      mask Display:
      | image(imread('sm_stewart_platform_hexagonplate.png'))
      | color('white')
      | port_label('LConn', 1, 'ref')
      | port_label('RConn', 1, 'leg1')
      | port_label('RConn', 2, 'leg2')
      | port_label('RConn', 3, 'leg3')
      | port_label('RConn', 4, 'leg4')
      | port_label('RConn', 5, 'leg5')
      | port_label('RConn', 6, 'leg6')
      | port_label('Output', 1, 'plat_ang')
  Solver Configuration : nesl_utility/Solver Configuration  PhysicalDomain=network_engine_domain  SubClassName=solver  LeftPortType=input  RightPortType=generic  Tones=[]  Harmonics=[]  SimulateNoise=off  Profile=off  UseLocalSampling=off  EnableSwitchedLinearOptims=on  FrequencyDomain=off  UseCCode=off  RelTol=0.001  AbsTol=1e-06  MinStep=1e-09  ToWorkspace=off  RevertToSquareIcSolve=off  NumHomotopyIterations=100  PhasorMode=off  PhasorModeNumHarmonics=1  DoDC=off  ResidualTolerance=1e-9  UseLocalSolver=off  LocalSolverChoice=NE_BACKWARD_EULER_ADVANCER  LocalSolverSampleTime=.001  DoFixedCost=off  MaxNonlinIter=3  MaxModeIter=2  LinearAlgebra=Sparse  EquationFormulation=NE_TIME_EF  DelaysMemoryBudget=1024  AutomaticFiltering=on  FilteringTimeConstant=0.001  PartitionStorageMethod=AS_NEEDED  PartitionMemoryBudget=1024  PartitionMethod=FAST
  World Frame : sm_lib/Frames and Transforms/World Frame
  world : PMIOPort  Side=Left
  gripper : PMIOPort  Port=2  Side=Right
  pos : Outport  VectorParamsAs1DForOutWhenUnconnected=off
  vel : Outport  Port=2  VectorParamsAs1DForOutWhenUnconnected=off
  acc : Outport  Port=3  VectorParamsAs1DForOutWhenUnconnected=off
  base_ang_from_leg : Outport  Port=4  VectorParamsAs1DForOutWhenUnconnected=off
  plat_ang : Outport  Port=5  VectorParamsAs1DForOutWhenUnconnected=off
  plat_ang_from_leg : Outport  Port=6  VectorParamsAs1DForOutWhenUnconnected=off
  base_ang : Outport  Port=7  VectorParamsAs1DForOutWhenUnconnected=off
  wires:
  Demux/1 -> [F1]
  Demux/2 -> [F2]
  Demux/3 -> [F3]
  Demux/4 -> [F4]
  Demux/5 -> [F5]
  Demux/6 -> [F6]
  [F1] -> Leg 1/1
  [F2] -> Leg 2/1
  [F3] -> Leg 3/1
  [F4] -> Leg 4/1
  [F5] -> Leg 5/1
  [F6] -> Leg 6/1
  force/1 -> Demux/1
  Leg 1/1 -> [P1]
  Leg 1/2 -> [V1]
  Leg 2/1 -> [P2]
  Leg 2/2 -> [V2]
  Leg 3/1 -> [P3]
  Leg 3/2 -> [V3]
  Leg 4/1 -> [P4]
  Leg 4/2 -> [V4]
  Leg 5/1 -> [P5]
  Leg 5/2 -> [V5]
  Leg 6/1 -> [P6]
  Leg 6/2 -> [V6]
  Mux/1 -> pos/1
  [P1] -> Mux/1
  [P2] -> Mux/2
  [P3] -> Mux/3
  [P4] -> Mux/4
  [P5] -> Mux/5
  [P6] -> Mux/6
  [V1] -> Mux1/1
  [V2] -> Mux1/2
  [V3] -> Mux1/3
  [V4] -> Mux1/4
  [V5] -> Mux1/5
  [V6] -> Mux1/6
  Mux1/1 -> vel/1
  [A6] -> Mux2/6
  Mux2/1 -> acc/1
  [A1] -> Mux2/1
  [A4] -> Mux2/4
  [A2] -> Mux2/2
  [A3] -> Mux2/3
  [A5] -> Mux2/5
  Leg 1/3 -> [A1]
  [B4] -> Mux3/4
  [B2] -> Mux3/2
  Mux3/1 -> base_ang_from_leg/1
  [B6] -> Mux3/6
  [B3] -> Mux3/3
  [B5] -> Mux3/5
  [B1] -> Mux3/1
  [T4] -> Mux4/4
  [T2] -> Mux4/2
  [T6] -> Mux4/6
  [T3] -> Mux4/3
  [T5] -> Mux4/5
  [T1] -> Mux4/1
  Leg 1/4 -> [B1]
  Leg 1/5 -> [T1]
  Leg 2/3 -> [A2]
  Leg 2/4 -> [B2]
  Leg 2/5 -> [T2]
  Leg 3/3 -> [A3]
  Leg 3/4 -> [B3]
  Leg 3/5 -> [T3]
  Leg 4/3 -> [A4]
  Leg 4/4 -> [B4]
  Leg 4/5 -> [T4]
  Leg 5/3 -> [A5]
  Leg 5/4 -> [B5]
  Leg 5/5 -> [T5]
  Leg 6/3 -> [A6]
  Leg 6/4 -> [B6]
  Leg 6/5 -> [T6]
  Platform/1(plat_ang) -> plat_ang/1
  Mux4/1 -> plat_ang_from_leg/1
  Base/1(ang) -> base_ang/1
  connections:
  Platform/LConn1 -- gripper/RConn1 -- Solver Configuration/RConn1
  Mechanism Configuration/RConn1 -- Base/LConn1 -- World Frame/RConn1 -- world/RConn1
  Leg 1/LConn1 -- Base/RConn1
  Leg 1/RConn1 -- Platform/RConn1
  Leg 2/LConn1 -- Base/RConn2
  Leg 2/RConn1 -- Platform/RConn2
  Leg 3/LConn1 -- Base/RConn3
  Leg 3/RConn1 -- Platform/RConn3
  Base/RConn4 -- Leg 4/LConn1
  Leg 4/RConn1 -- Platform/RConn4
  Leg 5/LConn1 -- Base/RConn5
  Leg 5/RConn1 -- Platform/RConn5
  Platform/RConn6 -- Leg 6/RConn1
  Base/RConn6 -- Leg 6/LConn1
